simulink model "test1"  (R2022b)
settings: Solver=VariableStepAuto  StartTime=0.0  StopTime=5  RelTol=1e-3
undefined symbols (not defined in the file): F, Light, MIL
libraries: shared6dof x1, aerolibwind2 x1, sharedtransform x1
settings Model: Creator=david  LastModifiedBy=david

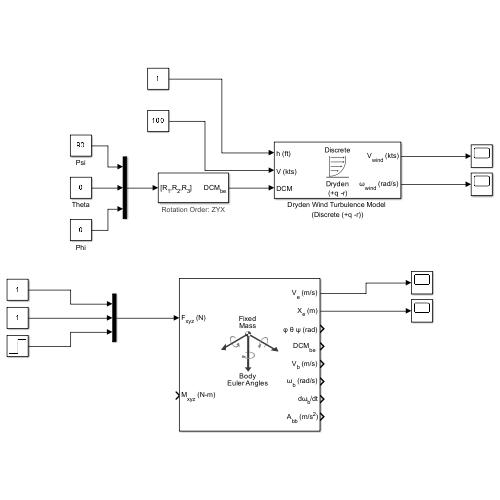
[thumbnail: Simulink's stored preview of the top-level diagram]
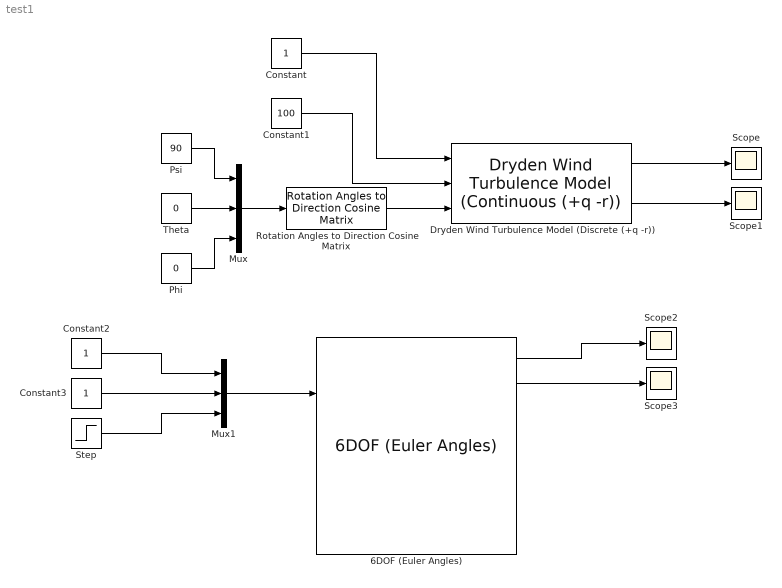
== system test1 ==
  6DOF (Euler Angles) : shared6dof/6DOF (Euler Angles)  units=Metric (MKS)  mtype=Fixed  rep=Euler Angles  xme_0=[0 0 0]  Vm_0=[0 0 0]  eul_0=[0 0 0]  pm_0=[0 0 0]  mass_0=1.0  mass_e=0.5  mass_f=2.0  inertia=eye(3)  inertia_e=eye(3)  inertia_f=2*eye(3)  k_quat=1.0  vre_flag=on  abi_flag=off  aMode=0  xme_statename=''  Vm_statename=''  eul_statename=''  quat_statename=''  pm_statename=''  mass_statename=''
  Constant : Constant
  Constant1 : Constant  Value=100
  Constant2 : Constant
  Constant3 : Constant
  Dryden Wind Turbulence Model (Discrete (+q -r)) : aerolibwind2/Dryden Wind Turbulence Model  (Continuous (+q -r))  units=English (Velocity in kts)  spec=MIL-F-8785C  model=Discrete Dryden (+q -r)  W20=15  Wdeg=0  TurbProb=10^-2 - Light  L_high=533.4  Wingspan=10  ts=0.1  Seed=[23341 23342 23343 23344]  T_on=on
      settings: LibrarySourceBlock=|
      | aerolibwind2/Dryden Wind Turbulence Model
      | (Discrete (+q -r))
  Mux : Mux  Inputs=3
  Mux1 : Mux  Inputs=3
  Phi : Constant  Value=0
  Psi : Constant  Value=90
  Rotation Angles to Direction Cosine Matrix : sharedtransform/Rotation Angles to Direction Cosine Matrix  rotationOrder=ZYX  aMode=aMode
  Scope{,1..3} (4 alike) : Scope
  Step : Step  After=100  SampleTime=0
  Theta : Constant  Value=0
  wires:
  Psi/1 -> Mux/1
  Theta/1 -> Mux/2
  Phi/1 -> Mux/3
  Dryden Wind Turbulence Model (Discrete (+q -r))/1 -> Scope/1
  Constant/1 -> Dryden Wind Turbulence Model (Discrete (+q -r))/1
  Constant1/1 -> Dryden Wind Turbulence Model (Discrete (+q -r))/2
  Mux/1 -> Rotation Angles to Direction Cosine Matrix/1
  Rotation Angles to Direction Cosine Matrix/1 -> Dryden Wind Turbulence Model (Discrete (+q -r))/3
  Dryden Wind Turbulence Model (Discrete (+q -r))/2 -> Scope1/1
  Step/1 -> Mux1/3
  Mux1/1 -> 6DOF (Euler Angles)/1
  Constant3/1 -> Mux1/2
  Constant2/1 -> Mux1/1
  6DOF (Euler Angles)/1 -> Scope2/1
  6DOF (Euler Angles)/2 -> Scope3/1
